simulink model "test_model"  (R2023b)
settings: Solver=VariableStepAuto  StartTime=0.0  StopTime=10.0  RelTol=1e-3
settings Model: Creator=hdt  LastModifiedBy=hdt

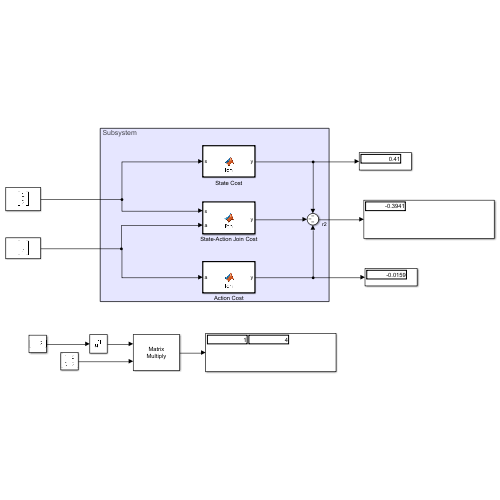
[thumbnail: Simulink's stored preview of the top-level diagram]
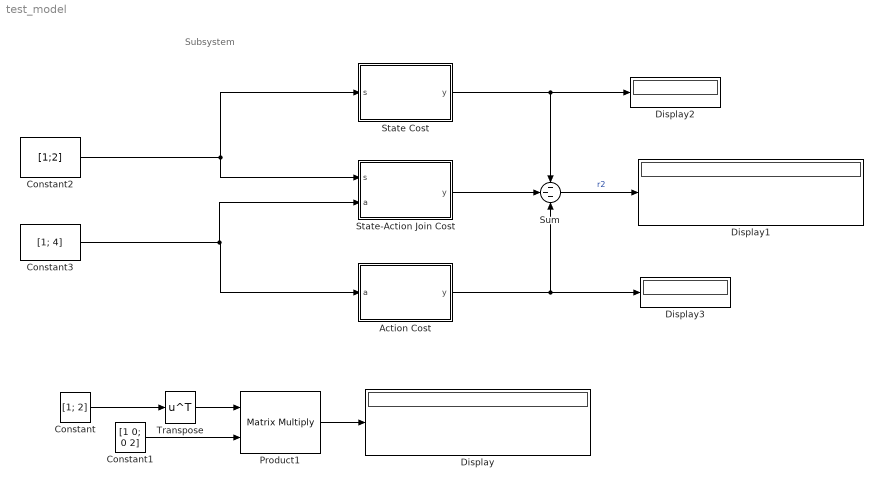
== system test_model ==
  note: Subsystem
  Action Cost : MATLAB Function  TreatAsAtomicUnit=on
  Constant : Constant  Value=[1; 2]
  Constant1 : Constant  Value=[1 0; 0 2]
  Constant2 : Constant  Value=[1;2]  VectorParams1D=off
  Constant3 : Constant  Value=[1; 4]  VectorParams1D=off
  Display{,1..3} (4 alike) : Display
  Product1 : Product  Multiplication=Matrix(*)
  State Cost : MATLAB Function  TreatAsAtomicUnit=on
  State-Action Join Cost : MATLAB Function  TreatAsAtomicUnit=on
  Sum : Sum  Inputs=---
  Transpose : Math  Operator=transpose
  wires:
  Constant/1 -> Transpose/1
  Product1/1 -> Display/1
  Constant1/1 -> Product1/2
  Transpose/1 -> Product1/1
  State Cost/1(y) -> Display2/1, Sum/1
  Sum/1 -> Display1/1  "r2"
  Action Cost/1(y) -> Display3/1, Sum/3
  State-Action Join Cost/1(y) -> Sum/2
  Constant3/1 -> State-Action Join Cost/2(a), Action Cost/1(a)
  Constant2/1 -> State Cost/1(s), State-Action Join Cost/1(s)

== matlab function test_model/State Cost ==
  data: s input; y output
function y = fcn(s)
    y = s'*QuadraticGains.Q*s;
end

== matlab function test_model/State-Action Join Cost ==
  data: s input; a input; y output
function y = fcn(s, a)
    y = 2*s'*QuadraticGains.N*a;
end

== matlab function test_model/Action Cost ==
  data: a input; y output
function y = fcn(a)
    y = a'*QuadraticGains.R*a;
end
